simulink model "lab02es2"  (R2021b)
settings: Solver=VariableStepAuto  StartTime=0.0  StopTime=200  RelTol=1e-3
undefined symbols (not defined in the file): exprnd, m, n
libraries: fl_lib x1
settings Model: Creator=francescafornasier  LastModifiedBy=francescafornasier

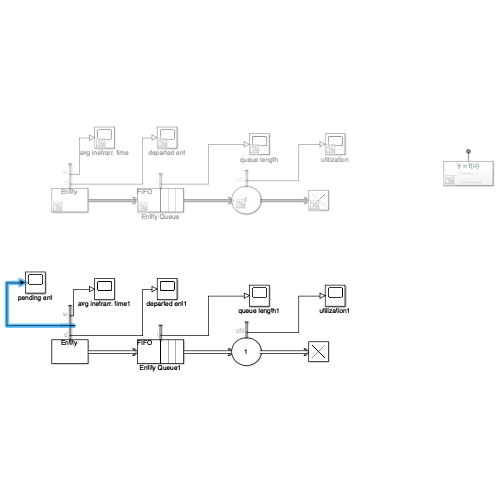
[thumbnail: Simulink's stored preview of the top-level diagram]
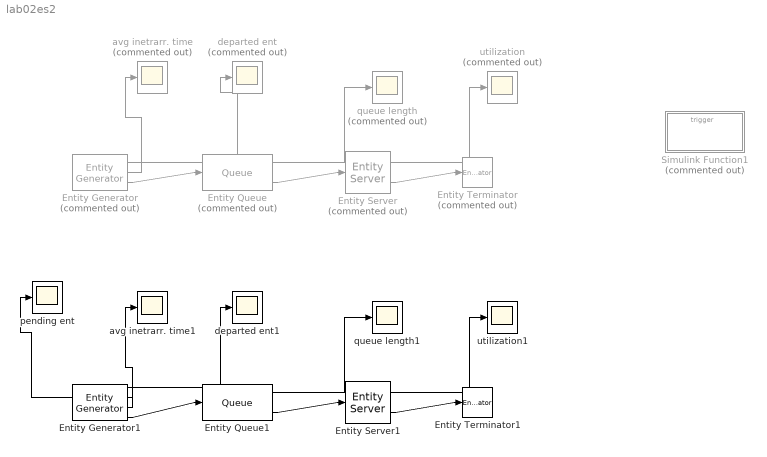
== system lab02es2 ==
  Entity Generator : EntityGenerator  Commented=on  OutputPortMessageModes=n,n,m  TimeSource=MATLAB action  IntergenerationTimeAction=dt = exprnd(2);  GenerateEntityAtSimulationStart=off  NumberEntitiesDeparted=on  AverageIntergenerationTime=on  EntityType=Structured  EntityTypeName=Entity
      settings: OutputPortMap=o0,o2,o3
  Entity Generator1 : EntityGenerator  OutputPortMessageModes=n,n,n,m  TimeSource=MATLAB action  IntergenerationTimeAction=dt = exprnd(2);  GenerateEntityAtSimulationStart=off  NumberEntitiesDeparted=on  PendingEntityInBlock=on  AverageIntergenerationTime=on  EntityType=Structured  EntityTypeName=Entity
      settings: OutputPortMap=o0,o1,o2,o3
  Entity Queue : Queue  Commented=on  InputPortMessageModes=m  OutputPortMessageModes=n,m  Capacity=inf  AverageQueueLength=on
      settings: OutputPortMap=o3,o5
  Entity Queue1 : Queue  InputPortMessageModes=m  OutputPortMessageModes=n,m  Capacity=5  AverageQueueLength=on
      settings: OutputPortMap=o3,o5
  Entity Server : EntityServer  Commented=on  InputPortMessageModes=m  OutputPortMessageModes=n,m  Capacity=1  ServiceTimeSource=MATLAB action  ServiceTimeValue=exprnd(1)  ServiceTimeAction=dt = exprnd(1);  Utilization=on
      settings: OutputPortMap=o5,o9
  Entity Server1 : EntityServer  InputPortMessageModes=m  OutputPortMessageModes=n,m  Capacity=1  ServiceTimeSource=MATLAB action  ServiceTimeValue=exprnd(1)  ServiceTimeAction=dt = exprnd(1);  Utilization=on
      settings: OutputPortMap=o5,o9
  Entity Terminator : EntityTerminator  Commented=on  InputPortMessageModes=m
  Entity Terminator1 : EntityTerminator  InputPortMessageModes=m
  Simulink Function1 : Subsystem  Commented=on  TreatAsAtomicUnit=on
  avg inetrarr. time : Scope  Commented=on
  avg inetrarr. time1 : Scope
  departed ent : Scope  Commented=on
  departed ent1 : Scope
  pending ent : Scope
  queue length : Scope  Commented=on
  queue length1 : Scope
  utilization : Scope  Commented=on
  utilization1 : Scope
  wires:
  Entity Generator/3 -> Entity Queue/1
  Entity Queue/2 -> Entity Server/1
  Entity Server/2 -> Entity Terminator/1
  Entity Generator/2 -> avg inetrarr. time/1
  Entity Generator/1 -> departed ent/1
  Entity Queue/1 -> queue length/1
  Entity Server/1 -> utilization/1
  Entity Server1/2 -> Entity Terminator1/1
  Entity Queue1/2 -> Entity Server1/1
  Entity Generator1/3 -> avg inetrarr. time1/1
  Entity Generator1/1 -> departed ent1/1
  Entity Generator1/4 -> Entity Queue1/1
  Entity Queue1/1 -> queue length1/1
  Entity Server1/1 -> utilization1/1
  Entity Generator1/2 -> pending ent/1

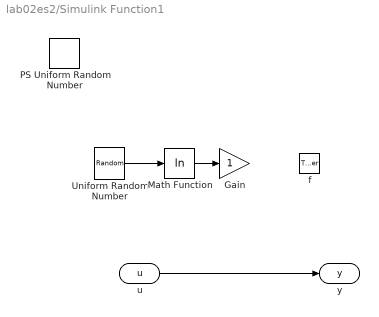
== system lab02es2/Simulink Function1 ==
  f : TriggerPort  TriggerType=function-call  IsSimulinkFunction=on  FunctionName=f  FunctionVisibility=scoped  VariantControl=(inherit)
  Gain : Gain
  Math Function : Math  Operator=log  SaturateOnIntegerOverflow=on
  PS Uniform Random Number : fl_lib/Physical Signals/Sources/PS Uniform Random Number  minimum=0  maximum=1  initial_seed=0  sample_time=1 s
      settings: SourceProductBaseCode=SS  InternalSimscapePortConfiguration="{\"Bottom\":[],\"Left\":[],\"Right\":[{\"id\":\"Y\",\"label\":\"Y\",\"type\":\"output\"}],\"Top\":[]}"
  Uniform Random Number : UniformRandomNumber  SampleTime=0.1
  u : ArgIn  DisableCoverage=on  ArgumentName=u
  y : ArgOut  DisableCoverage=on  ArgumentName=y
  wires:
  u/1 -> y/1
  Uniform Random Number/1 -> Math Function/1
  Math Function/1 -> Gain/1
